simulink model "AC_drone_Simulation"  (R2014a)
settings: Solver=ode45  StartTime=0  StopTime=10  FixedStep=0.02  MaxStep=0.06  RelTol=1e-3
model workspace (MAT data in the model file):
  Sig = Simulink.Signal
  Sig.DataType = 'auto'
  Sig.Dimensions = -1
  Sig.DimensionsMode = 'auto'
  Sig.Complexity = 'auto'
  Sig.SampleTime = -1
  Sig.SamplingMode = 'auto'
Description:
  | This is a configurable quadcopter simulation.
  | This Simulink model demonstates attitude control.
  | 
  | Additional quadcopter modeling and simulation materials available at:
  | github.com/dch33/Quad-Sim
  | 
  | Copyright (C) 2014 D. Hartman, K. Landis, S. Moreno, J. Kim, M. Mehrer
  | 
  | License:
  |     This program is free software: you can redistribute it and/or modify
  |     it under the terms of the GNU LESSER GENERAL PUBLIC LICENSE as published by
  |     the Free Software Foundation, either version 3 of the License, or
  |     (at your option) any later version.
  | 
  |     This program is distributed in the hope that it will be useful,
  |     but WITHOUT ANY WARRANTY; without even the implied warranty of
  |     MERCHANTABILITY or FITNESS FOR A PARTICULAR PURPOSE.  See the
  |     GNU General Public License for more details.
  | 
  |     You should have received a copy of the GNU LESSER GENERAL PUBLIC LICENSE
  |     along with this program.  If not, see <http://www.gnu.org/licenses/>.
settings Model: ModifiedComment=khsun -- Fri Dec 16 20:50:28 2016 -- Version 1.117  Creator=David Hartman  LastModifiedBy=khsun
settings Model: ModifiedHistory=|
  | khsun -- Fri Dec 16 20:50:28 2016 -- Version 1.117
  | 
  | 
  | khsun -- Wed Dec 14 14:42:39 2016 -- Version 1.116
  | 
  | 
  | khsun -- Tue Dec 13 21:18:15 2016 -- Version 1.115
  | 
  | 
  | khsun -- Sat Dec 10 12:50:18 2016 -- Version 1.114
  | 
  | 
  | khsun -- Fri Dec 09 22:53:31 2016 -- Version 1.113
  | 
  | 
  | khsun -- Fri Dec 09 13:27:57 2016 -- Version 1.112
  | 
  | 
  | khsun -- Mon Dec 05 00:13:18 2016 -- Version 1.111
  | 
  | 
  | khsun -- Sun Dec 04 22:04:49 2016 -- Version 1.110
  | 
  | 
  | khsun -- Sun Dec 04 21:59:44 2016 -- Version 1.109
  | 
  | 
  | khsun -- Sun Dec 04 19:56:43 2016 -- Version 1.108
  | 
  | 
  | khsun -- Sun Dec 04 17:51:08 2016 -- Version 1.107
  | 
  | 
  | khsun -- Sun Dec 04 17:51:05 2016 -- Version 1.106
  | 
  | 
  | sstal -- Sun Dec 04 03:27:38 2016 -- Version 1.105
  | 
  | 
  | sstal -- Sun Dec 04 02:23:26 2016 -- Version 1.104
  | 
  | 
  | sstal -- Sun Dec 04 01:58:29 2016 -- Version 1.103
  | 
  | 
  | sstal -- Sun Dec 04 01:49:36 2016 -- Version 1.102
  | 
  | 
  | sstal -- Sat Dec 03 22:54:16 2016 -- Version 1.101
  | 
  | 
  | sstal -- Sat Dec 03 22:52:17 2016 -- Version 1.100
  | 
  | 
  | sstal -- Fri Dec 02 21:35:40 2016 -- Version 1.99
  | 
  | 
  | sstal -- Fri Dec 02 20:50:23 2016 -- Version 1.98
  | 
  | 
  | sstal -- Fri Dec 02 19:45:10 2016 -- Version 1.97
  | 
  | 
  | sstal -- Fri Dec 02 16:57:20 2016 -- Version 1.96
  | 
  | 
  | SKY 05 -- Fri Dec 02 00:32:51 2016 -- Version 1.95
  | 
  | 
  | SKY 05 -- Thu Dec 01 23:20:58 2016 -- Version 1.94
  | 
  | 
  | SKY 05 -- Thu Dec 01 12:57:28 2016 -- Version 1.93
  | 
  | 
  | SKY 05 -- Wed Nov 30 14:36:02 2016 -- Version 1.92
  | 
  | 
  | SKY 03 -- Tue Nov 29 23:04:25 2016 -- Version 1.91
  | 
  | 
  | SKY 03 -- Tue Nov 29 22:01:09 2016 -- Version 1.90
  | 
  | 
  | SKY 03 -- Tue Nov 29 21:15:44 2016 -- Version 1.89
  | 
  | 
  | SKY 03 -- Tue Nov 29 19:16:05 2016 -- Version 1.88
  | 
  | 
  | SKY 03 -- Tue Nov 29 18:05:54 2016 -- Version 1.87
  | 
  | 
  | SKY 03 -- Tue Nov 29 14:57:27 2016 -- Version 1.86
  | 
  | 
  | SKY 03 -- Tue Nov 29 14:50:24 2016 -- Version 1.85
  | 
  | 
  | SKY 03 -- Tue Nov 29 14:29:54 2016 -- Version 1.84
  | 
  | 
  | SKY 03 -- Tue Nov 29 14:29:26 2016 -- Version 1.83
  | 
  | 
  | SKY 03 -- Tue Nov 29 14:12:46 2016 -- Version 1.82
  | 
  | 
  | SKY 05 -- Tue Nov 29 01:43:26 2016 -- Version 1.81
  | 
  | 
  | SKY 05 -- Tue Nov 29 00:54:08 2016 -- Version 1.80
  | 
  | 
  | SKY 05 -- Tue Nov 29 00:24:35 2016 -- Version 1.79
  | 
  | 
  | SKY 05 -- Tue Nov 29 00:14:25 2016 -- Version 1.78
  | 
  | 
  | SKY 05 -- Tue Nov 29 00:11:46 2016 -- Version 1.77
  | 
  | 
  | SKY 05 -- Tue Nov 29 00:10:44 2016 -- Version 1.76
  | 
  | 
  | SKY 05 -- Mon Nov 28 23:29:36 2016 -- Version 1.75
  | 
  | 
  | SKY 05 -- Mon Nov 28 23:29:19 2016 -- Version 1.74
  | 
  | 
  | SKY 05 -- Mon Nov 28 23:23:54 2016 -- Version 1.73
  | 
  | 
  | SKY 05 -- Mon Nov 28 17:23:20 2016 -- Version 1.72
  | 
  | 
  | SKY 05 -- Mon Nov 28 15:05:10 2016 -- Version 1.71
  | 
  | 
  | SKY 05 -- Mon Nov 28 15:03:54 2016 -- Version 1.70
  | 
  | 
  | SKY 05 -- Mon Nov 28 15:01:18 2016 -- Version 1.69
  | 
  | 
  | SKY 05 -- Mon Nov 28 14:59:20 2016 -- Version 1.68
  | 
  | 
  | SKY15 -- Tue Dec 27 23:01:23 2016 -- Version 1.67
  | 
  | 
  | SKY 05 -- Sun Nov 27 00:40:54 2016 -- Version 1.66
  | 
  | 
  | SKY 05 -- Sun Nov 27 00:39:41 2016 -- Version 1.65
  | 
  | 
  | SKY 05 -- Sun Nov 27 00:35:40 2016 -- Version 1.64
  | 
  | 
  | SKY 05 -- Sun Nov 27 00:31:30 2016 -- Version 1.63
  | 
  | 
  | SKY 05 -- Sat Nov 26 23:45:19 2016 -- Version 1.62
  | 
  | 
  | SKY 05 -- Sat Nov 26 22:11:47 2016 -- Version 1.61
  | 
  | 
  | SKY 05 -- Sat Nov 26 22:06:18 2016 -- Version 1.60
  | 
  | 
  | SKY 05 -- Sat Nov 26 21:42:29 2016 -- Version 1.59
  | 
  | 
  | khsun -- Sat Nov 26 20:51:23 2016 -- Version 1.58
  | 
  | 
  | khsun -- Sat Nov 26 20:25:48 2016 -- Version 1.57
  | 
  | 
  | khsun -- Sat Nov 26 20:20:04 2016 -- Version 1.56
  | 
  | 
  | khsun -- Sat Nov 26 20:15:53 2016 -- Version 1.55
  | 
  | 
  | khsun -- Sat Nov 26 19:10:38 2016 -- Version 1.54
  | 
  | 
  | khsun -- Sat Nov 26 18:25:01 2016 -- Version 1.53
  | 
  | 
  | khsun -- Sat Nov 26 17:24:24 2016 -- Version 1.52
  | 
  | 
  | khsun -- Sat Nov 26 17:17:34 2016 -- Version 1.51
  | 
  | 
  | khsun -- Sat Nov 26 16:55:15 2016 -- Version 1.50
  | 
  | 
  | khsun -- Sat Nov 26 16:52:55 2016 -- Version 1.49
  | 
  | 
  | khsun -- Sat Nov 26 16:49:39 2016 -- Version 1.48
  | 
  | 
  | khsun -- Sat Nov 26 16:21:13 2016 -- Version 1.47
  | 
  | 
  | khsun -- Sat Nov 26 16:21:01 2016 -- Version 1.46
  | 
  | 
  | khsun -- Sat Nov 26 16:20:27 2016 -- Version 1.45
  | 
  | 
  | khsun -- Sat Nov 26 12:23:16 2016 -- Version 1.44
  | 
  | 
  | khsun -- Sat Nov 26 12:22:44 2016 -- Version 1.43
  | 
  | 
  | khsun -- Sat Nov 26 12:09:40 2016 -- Version 1.42
  | 
  | 
  | khsun -- Fri Nov 25 12:53:36 2016 -- Version 1.41
  | 
  | 
  | khsun -- Thu Nov 24 15:51:55 2016 -- Version 1.40
  | 
  | 
  | khsun -- Thu Nov 24 15:40:52 2016 -- Version 1.39
  | 
  | 
  | khsun -- Thu Nov 24 15:25:38 2016 -- Version 1.38
  | 
  | 
  | khsun -- Thu Nov 24 15:20:43 2016 -- Version 1.37
  | 
  | 
  | khsun -- Thu Nov 24 15:15:05 2016 -- Version 1.36
  | 
  | 
  | khsun -- Thu Nov 24 15:14:02 2016 -- Version 1.35
  | 
  | 
  | khsun -- Thu Nov 24 11:17:00 2016 -- Version 1.34
  | 
  | 
  | khsun -- Wed Nov 23 23:17:43 2016 -- Version 1.33
  | 
  | 
  | khsun -- Wed Nov 23 17:41:56 2016 -- Version 1.31
  | 
  | 
  | khsun -- Wed Nov 23 17:41:56 2016 -- Version 1.31
  | 
  | 
  | khsun -- Tue Nov 22 22:20:06 2016 -- Version 1.30
  | 
  | 
  | khsun -- Tue Nov 22 22:09:32 2016 -- Version 1.29
  | 
  | 
  | khsun -- Tue Nov 22 22:08:32 2016 -- Version 1.28
  | 
  | 
  | khsun -- Tue Nov 22 22:07:24 2016 -- Version 1.27
  | 
  | 
  | khsun -- Tue Nov 22 22:06:29 2016 -- Version 1.26
  | 
  | 
  | khsun -- Tue Nov 22 22:06:06 2016 -- Version 1.25
  | 
  | 
  | khsun -- Tue Nov 22 22:03:53 2016 -- Version 1.24
  | 
  | 
  | khsun -- Tue Nov 22 21:01:42 2016 -- Version 1.23
  | 
  | 
  | khsun -- Tue Nov 22 20:59:39 2016 -- Version 1.22
  | 
  | 
  | khsun -- Tue Nov 22 20:24:50 2016 -- Version 1.21
  | 
  | 
  | khsun -- Tue Nov 22 20:14:42 2016 -- Version 1.20
  | 
  | 
  | khsun -- Tue Nov 22 16:24:10 2016 -- Version 1.19
  | 
  | 
  | khsun -- Tue Nov 22 16:10:18 2016 -- Version 1.18
  | 
  | 
  | khsun -- Tue Nov 22 11:35:43 2016 -- Version 1.17
  | 
  | 
  | khsun -- Tue Nov 22 10:54:15 2016 -- Version 1.16
  | 
  | 
  | khsun -- Mon Nov 21 21:57:53 2016 -- Version 1.15
  | 
  | 
  | khsun -- Mon Nov 21 21:12:45 2016 -- Version 1.14
  | 
  | 
  | khsun -- Sun Nov 20 22:34:28 2016 -- Version 1.13
  | 
  | 
  | khsun -- Sun Nov 20 19:39:17 2016 -- Version 1.12
  | 
  | 
  | khsun -- Sun Nov 20 17:26:15 2016 -- Version 1.11
  | 
  | 
  | khsun -- Sun Nov 20 17:01:09 2016 -- Version 1.10
  | 
  | 
  | khsun -- Sun Nov 20 15:27:38 2016 -- Version 1.9
  | 
  | 
  | khsun -- Sun Nov 20 15:24:18 2016 -- Version 1.8
  | 
  | 
  | khsun -- Sun Nov 20 15:24:12 2016 -- Version 1.7
  | 
  | 
  | khsun -- Sun Nov 20 14:36:24 2016 -- Version 1.6
  | 
  | 
  | davidhartman -- Fri Jun 06 23:19:51 2014 -- Version 1.5
  | 
  | 
  | davidhartman -- Fri Jun 06 22:53:10 2014 -- Version 1.3
settings SolverCC: AutoInsertRateTranBlk=on
settings DataIOCC: LimitDataPoints=off  SignalLogging=off
settings OptimizationCC: InlineParams=on
settings DebuggingCC: UnderspecifiedInitializationDetection=Classic  UniqueDataStoreMsg=warning  StateNameClashWarn=warning  StrictBusMsg=WarnOnBusTreatedAsVector

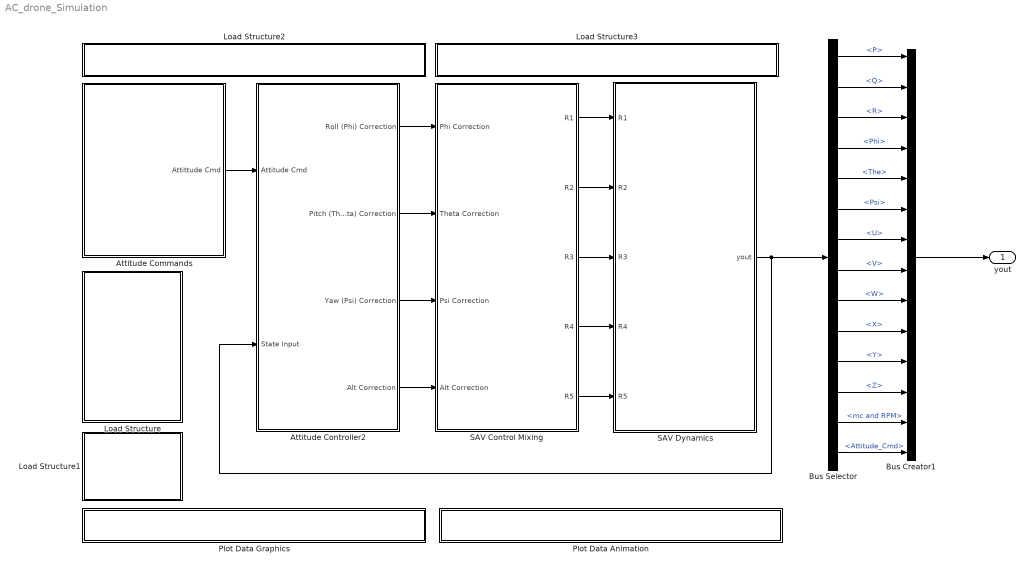
== system AC_drone_Simulation ==
  Attitude Commands : Subsystem
  Attitude Controller2 : Subsystem
  Bus Creator1 : BusCreator  Inputs='P','Q','R','Phi','The','Psi','U','V','W','X','Y','Z','mc and RPM','Attitude_Cmd'
  Bus Selector : BusSelector  OutputSignals=P,Q,R,Phi,The,Psi,U,V,W,X,Y,Z,mc and RPM,Attitude_Cmd
  Load Structure : Subsystem
      settings: OpenFcn=|
      | uiopen('load')
      | if (exist('IC')==1 && exist('quadModel')==1)
      | set_param(bdroot, 'SimulationCommand', 'update')
      | end
      mask Display: fprintf('LOAD:\nQuadcopter\nModel Or\nInitial\nConditions');
  Load Structure1 : Subsystem
      settings: OpenFcn=|
      | if (exist('IC')==1 && exist('quadModel')==1 && exist('yout') && exist('tout'))
      | saveSimResults()
      | else
      | msgbox('No Data To Save!')
      | end
      mask Display: fprintf('SAVE:\nSimulation\nResults');
  Load Structure2 : Subsystem
      settings: OpenFcn=|
      | if exist('GUI_Modeling') == 2,
      | run('GUI_Modeling')
      | 
      | else
      | 
      | msgbox('The desired GUI must be first added to MATLABs path.')
      | 
      | end
      mask Display: fprintf('OPEN GUI: Build New \n Model');
  Load Structure3 : Subsystem
      settings: OpenFcn=|
      | if exist('GUI_IC') == 2,
      | run('GUI_IC')
      | 
      | else
      | 
      | msgbox('The desired GUI must be first added to MATLABs path.')
      | 
      | end
      mask Display: fprintf('OPEN GUI: Create Initial \n Conditions');
  Plot Data Animation : Subsystem
      settings: OpenFcn=|
      | if exist('QuadAnim4') == 2,
      |     if exist('yout')
      | 	run('QuadAnim4');
      |     else
      |     msgbox('Simulation must be run before data can be plotted.');
      |     end
      | else                                                                          msgbox('The desired GUI must be first added to MATLABs path.')
      | end
      mask Display: fprintf('OPEN GUI: Flight Animation')
  Plot Data Graphics : Subsystem
      settings: OpenFcn=|
      | if exist('yout')
      | yout = evalin('base', 'yout');
      | tout = evalin('base', 'tout');
      | quadPlots(yout, tout)
      | else
      | msgbox('Simulation must be run before data can be plotted.')
      | end
      mask Display: fprintf('OPEN PLOT: State Data')
  SAV Control Mixing : Subsystem
  SAV Dynamics : Subsystem
  yout : Outport
  wires:
  SAV Control Mixing/1(R1) -> SAV Dynamics/1(R1)
  SAV Control Mixing/2(R2) -> SAV Dynamics/2(R2)
  SAV Control Mixing/3(R3) -> SAV Dynamics/3(R3)
  SAV Control Mixing/4(R4) -> SAV Dynamics/4(R4)
  Attitude Commands/1(Attittude Cmd) -> Attitude Controller2/1(Attitude Cmd)
  SAV Dynamics/1(yout) -> Bus Selector/1, Attitude Controller2/2(State Input)
  Attitude Controller2/3(Yaw (Psi) Correction) -> SAV Control Mixing/3(Psi Correction)
  Attitude Controller2/2(Pitch (Theta) Correction) -> SAV Control Mixing/2(Theta Correction)
  Attitude Controller2/1(Roll (Phi) Correction) -> SAV Control Mixing/1(Phi Correction)
  Attitude Controller2/4(Alt Correction) -> SAV Control Mixing/4(Alt Correction)
  SAV Control Mixing/5(R5) -> SAV Dynamics/5(R5)
  Bus Creator1/1 -> yout/1
  Bus Selector/14 -> Bus Creator1/14  "<Attitude_Cmd>"
  Bus Selector/13 -> Bus Creator1/13  "<mc and RPM>"
  Bus Selector/12 -> Bus Creator1/12  "<Z>"
  Bus Selector/11 -> Bus Creator1/11  "<Y>"
  Bus Selector/10 -> Bus Creator1/10  "<X>"
  Bus Selector/9 -> Bus Creator1/9  "<W>"
  Bus Selector/8 -> Bus Creator1/8  "<V>"
  Bus Selector/7 -> Bus Creator1/7  "<U>"
  Bus Selector/6 -> Bus Creator1/6  "<Psi>"
  Bus Selector/5 -> Bus Creator1/5  "<The>"
  Bus Selector/4 -> Bus Creator1/4  "<Phi>"
  Bus Selector/3 -> Bus Creator1/3  "<R>"
  Bus Selector/2 -> Bus Creator1/2  "<Q>"
  Bus Selector/1 -> Bus Creator1/1  "<P>"

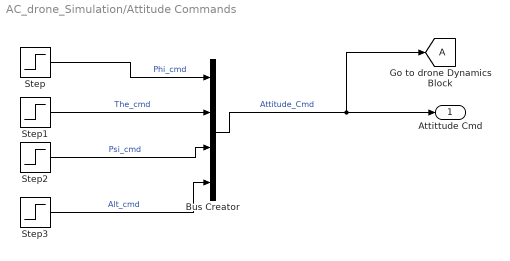
== system AC_drone_Simulation/Attitude Commands ==
  Bus Creator : BusCreator
  Step : Step  Time=0  After=0  SampleTime=0
  Step1 : Step  Time=0  After=20*pi/180  SampleTime=0
  Step2 : Step  Time=0  After=20*pi/180  SampleTime=0
  Step3 : Step  Time=0  Before=10  After=20  SampleTime=0
  Attittude Cmd : Outport
  tag scope: A=global
  wires:
  Bus Creator/1 -> Attittude Cmd/1, [A]  "Attitude_Cmd"
  Step1/1 -> Bus Creator/2  "The_cmd"
  Step/1 -> Bus Creator/1  "Phi_cmd"
  Step3/1 -> Bus Creator/4  "Alt_cmd"
  Step2/1 -> Bus Creator/3  "Psi_cmd"

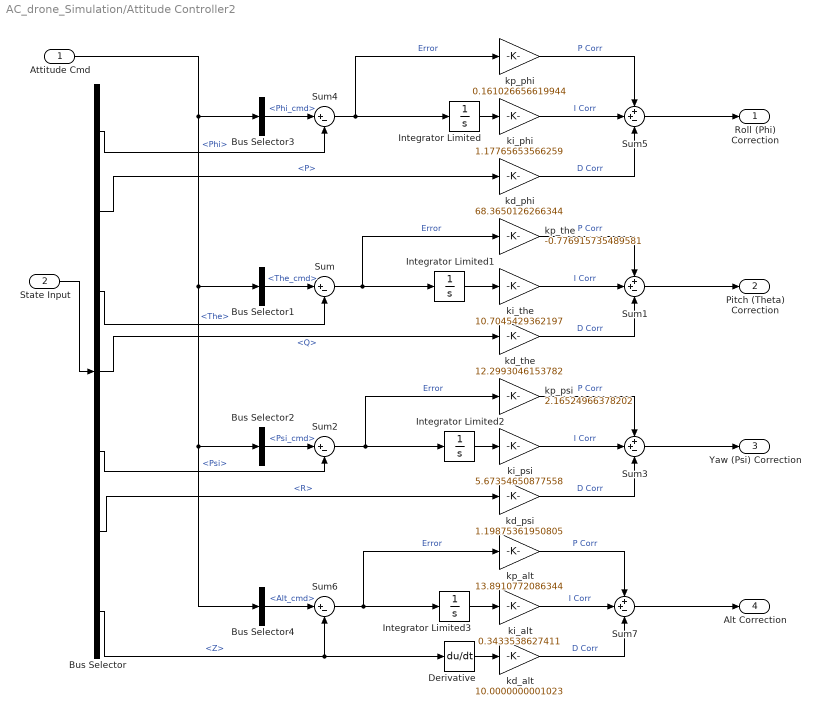
== system AC_drone_Simulation/Attitude Controller2 ==
  Attitude Cmd : Inport
  State Input : Inport  Port=2
  Bus Selector : BusSelector  OutputSignals=Phi,P,The,Q,Psi,R,Z
  Bus Selector1 : BusSelector  OutputSignals=The_cmd
  Bus Selector2 : BusSelector  OutputSignals=Psi_cmd
  Bus Selector3 : BusSelector  OutputSignals=Phi_cmd
  Bus Selector4 : BusSelector  OutputSignals=Alt_cmd
  Derivative : Derivative
  Integrator Limited{,1..3} (4 alike) : Integrator  LimitOutput=on  UpperSaturationLimit=1  LowerSaturationLimit=-1
  Sum{,2,4,6} (4 alike) : Sum  Inputs=|+-
  Sum{1,3,5,7} (4 alike) : Sum  Inputs=++-
  kd_alt : Gain  Gain=10.0000000001023
  kd_phi : Gain  Gain=68.3650126266344
  kd_psi : Gain  Gain=1.19875361950805
  kd_the : Gain  Gain=12.2993046153782
  ki_alt : Gain  Gain=0.3433538627411
  ki_phi : Gain  Gain=1.17765653566259
  ki_psi : Gain  Gain=5.67354650877558
  ki_the : Gain  Gain=10.7045429362197
  kp_alt : Gain  Gain=13.8910772086344
  kp_phi : Gain  Gain=0.161026656619944
  kp_psi : Gain  Gain=2.16524966378202
  kp_the : Gain  Gain=-0.776915735489581
  Roll (Phi) Correction : Outport
  Pitch (Theta) Correction : Outport  Port=2
  Yaw (Psi) Correction : Outport  Port=3
  Alt Correction : Outport  Port=4
  wires:
  Bus Selector/3 -> Sum/2  "<The>"
  Attitude Cmd/1 -> Bus Selector4/1, Bus Selector2/1, Bus Selector1/1, Bus Selector3/1
  Bus Selector/5 -> Sum2/2  "<Psi>"
  State Input/1 -> Bus Selector/1
  Bus Selector/1 -> Sum4/2  "<Phi>"
  Bus Selector/2 -> kd_phi/1  "<P>"
  Bus Selector/4 -> kd_the/1  "<Q>"
  Bus Selector/6 -> kd_psi/1  "<R>"
  Bus Selector1/1 -> Sum/1  "<The_cmd>"
  kd_the/1 -> Sum1/3  "D Corr"
  kp_the/1 -> Sum1/1  "P Corr"
  Sum1/1 -> Pitch (Theta) Correction/1
  Bus Selector2/1 -> Sum2/1  "<Psi_cmd>"
  kd_psi/1 -> Sum3/3  "D Corr"
  kp_psi/1 -> Sum3/1  "P Corr"
  Bus Selector3/1 -> Sum4/1  "<Phi_cmd>"
  kp_phi/1 -> Sum5/1  "P Corr"
  Sum5/1 -> Roll (Phi) Correction/1
  kd_phi/1 -> Sum5/3  "D Corr"
  Derivative/1 -> kd_alt/1
  Bus Selector4/1 -> Sum6/1  "<Alt_cmd>"
  kd_alt/1 -> Sum7/3  "D Corr"
  kp_alt/1 -> Sum7/1  "P Corr"
  Sum7/1 -> Alt Correction/1
  Bus Selector/7 -> Sum6/2, Derivative/1  "<Z>"
  Integrator Limited/1 -> ki_phi/1
  ki_phi/1 -> Sum5/2  "I Corr"
  Sum4/1 -> kp_phi/1, Integrator Limited/1  "Error"
  Integrator Limited1/1 -> ki_the/1
  ki_the/1 -> Sum1/2  "I Corr"
  Sum/1 -> kp_the/1, Integrator Limited1/1  "Error"
  Sum3/1 -> Yaw (Psi) Correction/1
  Integrator Limited2/1 -> ki_psi/1
  ki_psi/1 -> Sum3/2  "I Corr"
  Sum2/1 -> kp_psi/1, Integrator Limited2/1  "Error"
  Integrator Limited3/1 -> ki_alt/1
  ki_alt/1 -> Sum7/2  "I Corr"
  Sum6/1 -> kp_alt/1, Integrator Limited3/1  "Error"

== system AC_drone_Simulation/Load Structure ==

== system AC_drone_Simulation/Load Structure1 ==

== system AC_drone_Simulation/Load Structure2 ==

== system AC_drone_Simulation/Load Structure3 ==

== system AC_drone_Simulation/Plot Data Animation ==

== system AC_drone_Simulation/Plot Data Graphics ==

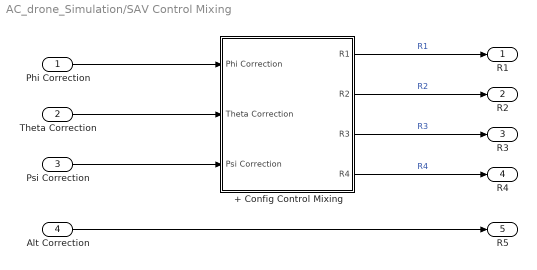
== system AC_drone_Simulation/SAV Control Mixing ==
  Phi Correction : Inport
  Theta Correction : Inport  Port=2
  Psi Correction : Inport  Port=3
  Alt Correction : Inport  Port=4
  + Config Control Mixing : Subsystem
  R1 : Outport
  R2 : Outport  Port=2
  R3 : Outport  Port=3
  R4 : Outport  Port=4
  R5 : Outport  Port=5
  wires:
  + Config Control Mixing/4(R4) -> R4/1  "R4"
  + Config Control Mixing/3(R3) -> R3/1  "R3"
  + Config Control Mixing/2(R2) -> R2/1  "R2"
  + Config Control Mixing/1(R1) -> R1/1  "R1"
  Psi Correction/1 -> + Config Control Mixing/3(Psi Correction)
  Theta Correction/1 -> + Config Control Mixing/2(Theta Correction)
  Phi Correction/1 -> + Config Control Mixing/1(Phi Correction)
  Alt Correction/1 -> R5/1

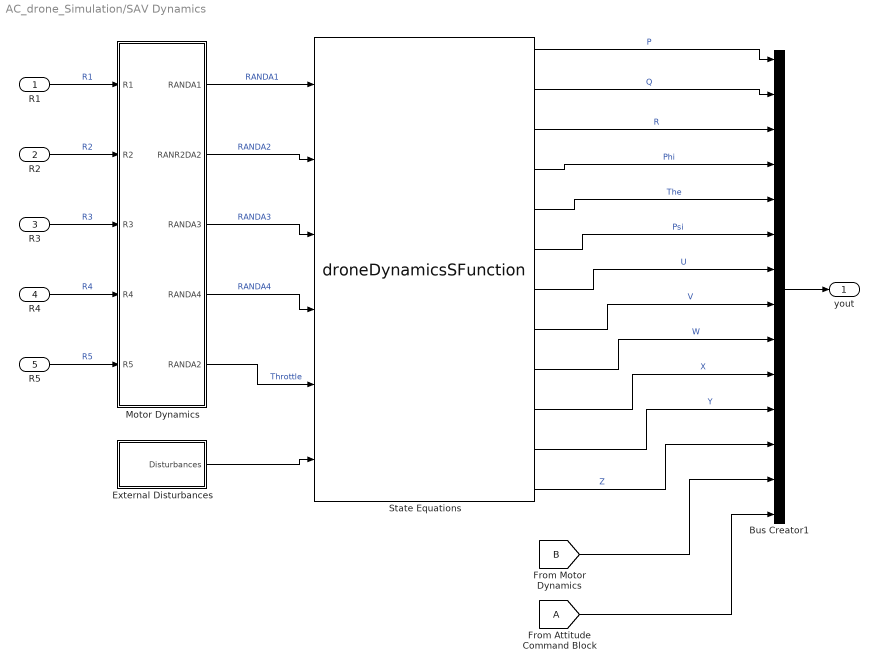
== system AC_drone_Simulation/SAV Dynamics ==
  R1 : Inport
  R2 : Inport  Port=2
  R3 : Inport  Port=3
  R4 : Inport  Port=4
  R5 : Inport  Port=5
  Bus Creator1 : BusCreator  Inputs='P','Q','R','Phi','The','Psi','U','V','W','X','Y','Z','mc and RPM','Attitude_Cmd'
  External Disturbances : Subsystem
  Motor Dynamics : Subsystem  mask{AOA=30*pi/180}
      mask prompts: AOA "Simulink:blkprm_prompts:SaturateUpLim"
      mask TypeOptions AOA: Signal_Saturation_1/UpperLimit | Signal_Saturation_2/UpperLimit | Signal_Saturation_3/UpperLimit | Signal_Saturation_4/UpperLimit
      mask Display: fprintf(['AOA = ' num2str(AOA*180/pi) '°']);
  State Equations : M-S-Function  FunctionName=droneDynamicsSFunction  Parameters=droneModel, IC
      mask Display:
      | port_label('input', 1, 'RANDA1')
      | port_label('input', 2, 'RANDA2')
      | port_label('input', 3, 'RANDA3')
      | port_label('input', 4, 'RANDA4')
      | port_label('input', 5, 'Throttle')
      | port_label('input', 6, 'Disturbances')
      | port_label('output', 1, 'P')
      | port_label('output', 2, 'Q')
      | port_label('output', 3, 'R')
      | port_label('output', 4, 'Phi')
      | port_label('output', 5, 'The')
      | port_label('output', 6, 'Psi')
      | port_label('output', 7, 'U')
      | port_label('output', 8, 'V')
      | port_label('output', 9, 'W')
      | port_label('output', 10, 'X')
      | port_label('output', 11, 'Y')
      | port_label('output', 12, 'Z')
  yout : Outport
  wires:
  [B] -> Bus Creator1/13
  [A] -> Bus Creator1/14
  R2/1 -> Motor Dynamics/2(R2)  "R2"
  R3/1 -> Motor Dynamics/3(R3)  "R3"
  R4/1 -> Motor Dynamics/4(R4)  "R4"
  R1/1 -> Motor Dynamics/1(R1)  "R1"
  Motor Dynamics/4(RANDA4) -> State Equations/4  "RANDA4"
  Motor Dynamics/3(RANDA3) -> State Equations/3  "RANDA3"
  Motor Dynamics/2(RANR2DA2) -> State Equations/2  "RANDA2"
  Motor Dynamics/1(RANDA1) -> State Equations/1  "RANDA1"
  State Equations/6 -> Bus Creator1/6  "Psi"
  State Equations/5 -> Bus Creator1/5  "The"
  State Equations/4 -> Bus Creator1/4  "Phi"
  State Equations/3 -> Bus Creator1/3  "R"
  State Equations/2 -> Bus Creator1/2  "Q"
  State Equations/1 -> Bus Creator1/1  "P"
  External Disturbances/1("Disturbances ") -> State Equations/6
  Bus Creator1/1 -> yout/1
  State Equations/12 -> Bus Creator1/12  "Z"
  State Equations/11 -> Bus Creator1/11  "Y"
  State Equations/10 -> Bus Creator1/10  "X"
  State Equations/9 -> Bus Creator1/9  "W"
  State Equations/7 -> Bus Creator1/7  "U"
  State Equations/8 -> Bus Creator1/8  "V"
  R5/1 -> Motor Dynamics/5(R5)  "R5"
  Motor Dynamics/5(RANDA2) -> State Equations/5  "Throttle"

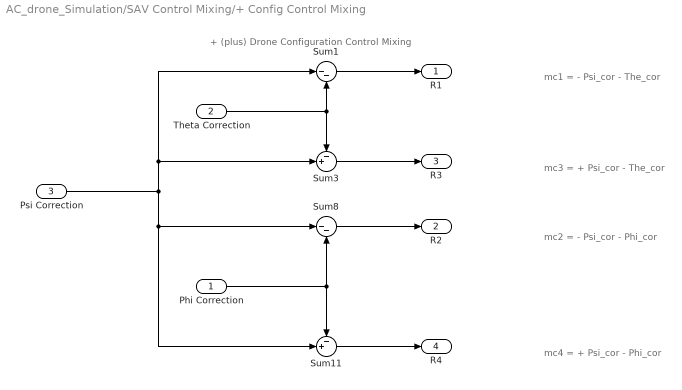
== system AC_drone_Simulation/SAV Control Mixing/+ Config Control Mixing ==
  note: mc1 = - Psi_cor - The_cor
  note: mc3 = + Psi_cor - The_cor
  note: mc4 = + Psi_cor - Phi_cor
  note: + (plus) Drone Configuration Control Mixing
  note: mc2 = - Psi_cor - Phi_cor
  Phi Correction : Inport
  Theta Correction : Inport  Port=2
  Psi Correction : Inport  Port=3
  Sum1 : Sum  Inputs=|--
  Sum11 : Sum  Inputs=-+|
  Sum3 : Sum  Inputs=-+|
  Sum8 : Sum  Inputs=|--
  R1 : Outport
  R2 : Outport  Port=2
  R3 : Outport  Port=3
  R4 : Outport  Port=4
  wires:
  Sum11/1 -> R4/1
  Sum8/1 -> R2/1
  Sum3/1 -> R3/1
  Sum1/1 -> R1/1
  Phi Correction/1 -> Sum11/1, Sum8/2
  Psi Correction/1 -> Sum11/2, Sum8/1, Sum1/1, Sum3/2
  Theta Correction/1 -> Sum3/1, Sum1/2

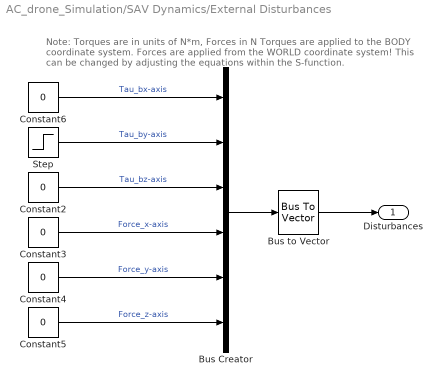
== system AC_drone_Simulation/SAV Dynamics/External Disturbances ==
  note: Note: Torques are in units of N*m, Forces in N
      | Torques are applied to the BODY coordinate system.
      | Forces are applied from the WORLD coordinate system!
      | This can be changed by adjusting the equations within the S-function.
  Bus Creator : BusCreator  Inputs=6
  Bus to Vector : BusToVector
  Constant{2..6} (5 alike) : Constant  Value=0
  Step : Step  Time=0  After=0  SampleTime=0
  "Disturbances " : Outport
  wires:
  Constant5/1 -> Bus Creator/6  "Force_z-axis"
  Constant4/1 -> Bus Creator/5  "Force_y-axis"
  Constant3/1 -> Bus Creator/4  "Force_x-axis"
  Constant2/1 -> Bus Creator/3  "Tau_bz-axis"
  Step/1 -> Bus Creator/2  "Tau_by-axis"
  Constant6/1 -> Bus Creator/1  "Tau_bx-axis"
  Bus Creator/1 -> Bus to Vector/1
  Bus to Vector/1 -> "Disturbances "/1

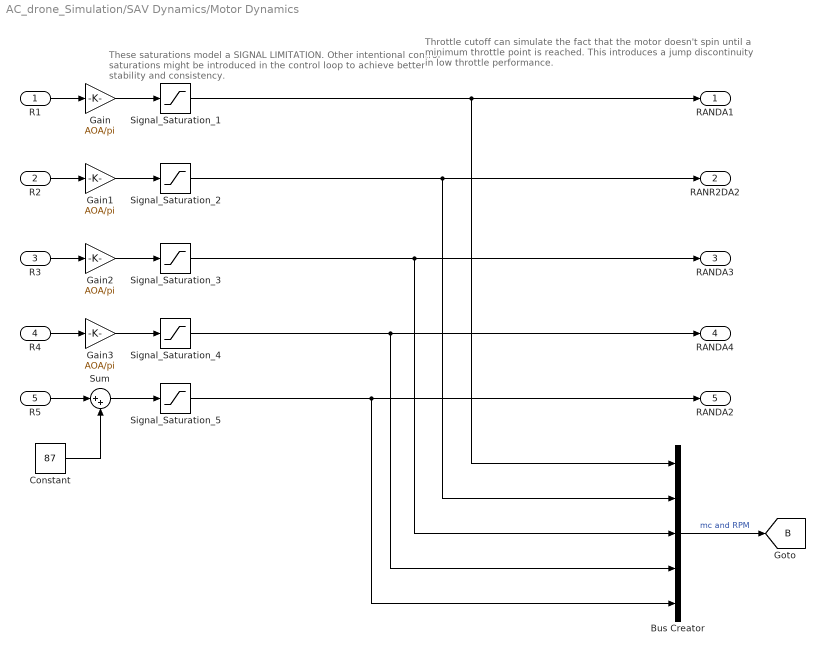
== system AC_drone_Simulation/SAV Dynamics/Motor Dynamics ==
  note: These saturations model a SIGNAL LIMITATION.
      | Other intentional control saturations might be introduced in the
      | control loop to achieve better stability and consistency.
  note: Throttle cutoff can simulate the fact that the motor doesn't
      | spin until a minimum throttle point is reached. This introduces
      | a jump discontinuity in low throttle performance.
  R1 : Inport
  R2 : Inport  Port=2
  R3 : Inport  Port=3
  R4 : Inport  Port=4
  R5 : Inport  Port=5
  Bus Creator : BusCreator  Inputs=5
  Constant : Constant  Value=87
  Gain{,1..3} (4 alike) : Gain  Gain=AOA/pi
  Signal_Saturation_{1..4} (4 alike) : Saturate  UpperLimit=AOA  LowerLimit=-AOA
  Signal_Saturation_5 : Saturate  UpperLimit=100  LowerLimit=64
  Sum : Sum  Inputs=|++
  RANDA1 : Outport
  RANR2DA2 : Outport  Port=2
  RANDA3 : Outport  Port=3
  RANDA4 : Outport  Port=4
  RANDA2 : Outport  Port=5
  tag scope: B=global
  wires:
  Bus Creator/1 -> [B]  "mc and RPM"
  Signal_Saturation_4/1 -> RANDA4/1, Bus Creator/4
  Signal_Saturation_3/1 -> RANDA3/1, Bus Creator/3
  Signal_Saturation_2/1 -> RANR2DA2/1, Bus Creator/2
  Signal_Saturation_1/1 -> RANDA1/1, Bus Creator/1
  R3/1 -> Gain2/1
  R2/1 -> Gain1/1
  R4/1 -> Gain3/1
  R1/1 -> Gain/1
  Gain/1 -> Signal_Saturation_1/1
  Gain1/1 -> Signal_Saturation_2/1
  Gain2/1 -> Signal_Saturation_3/1
  Gain3/1 -> Signal_Saturation_4/1
  R5/1 -> Sum/1
  Constant/1 -> Sum/2
  Sum/1 -> Signal_Saturation_5/1
  Signal_Saturation_5/1 -> RANDA2/1, Bus Creator/5
